simulink model "main_controller_sim"  (R2015a)
settings: Solver=ode45  StartTime=0.0  StopTime=10  FixedStep=1e-3  MaxStep=1e-3  RelTol=1e-3
values from neighbouring files (symbols this model uses):
  A = sys_rand.A    [main_Observer_states.m]
  B = B(:,1:end-1)    [main_Observer_states.m]
  beta = [5657.83678507 -1913.14902282 -932.285352789 348.153105943 2507.13858904 -2140.9545479]    [beta.mat]    (also in main_disturbance_observer.m = inv(delta2)*beta_hat)
  C = [0.617255113405149,0,0,-0.448535555941661,0.134230346538703,1.41932930409004;0.283640603624291,0,2.22808153625508,-1.86462753317668,-1.99763494036701,-0.0116516666362024;0.350975702033898,-0.174162030842294,1.44167650824058,-0.392420914284623,1.30288133017051,-0.392171726620127]    [finding_Y.m]    (also in main_Observer_states.m = sys_rand.C)
  Delta = (eye(n,n)+(-H*CHp+Y*(eye(p,p)-(C*H)*CHp))*C)*B    [main_Observer_states.m]    (also in observer.mat = [-0.0673817558455 0.158220969334 -1.63112233705 -0.121104966)
  Gama = eta*A-X*C    [main_Observer_states.m]    (also in observer.mat = [-0.665415381788 -1.71297839543 -11.0757301234 9.21615917151)
  H = B(:,end)    [main_Observer_states.m]
  Phi = dec2mat(LMISYS,xopt,2)    [main_Observer_states.m]    (also in observer.mat = [2.03974430811 -0.144807404976 -3.64797116197 7.53997403465 )
  theta = theta1+Y*theta2    [main_Observer_states.m]    (also in observer.mat = [-0.848682280391 0.936204937086 2.9983152382 2.21151006385 4)
  Tw = [0.110610315069 0.237446821355 -1.7873542646]    [Tw.mat]
  Tx = [0.778503771805 -0.0510386379765 1.1345792671 0.660349965935 0.317918162843 -0.19578141191 0.0703383785316 -0.0293855404701 0.00570882754881 0.572739299383 0.143983654558 -0.291796802072 ... (18 elements, 3x6)]    [Tx.mat]
libraries: simulink x1
settings Model: Creator=p4wp4w  LastModifiedBy=p4wp4w

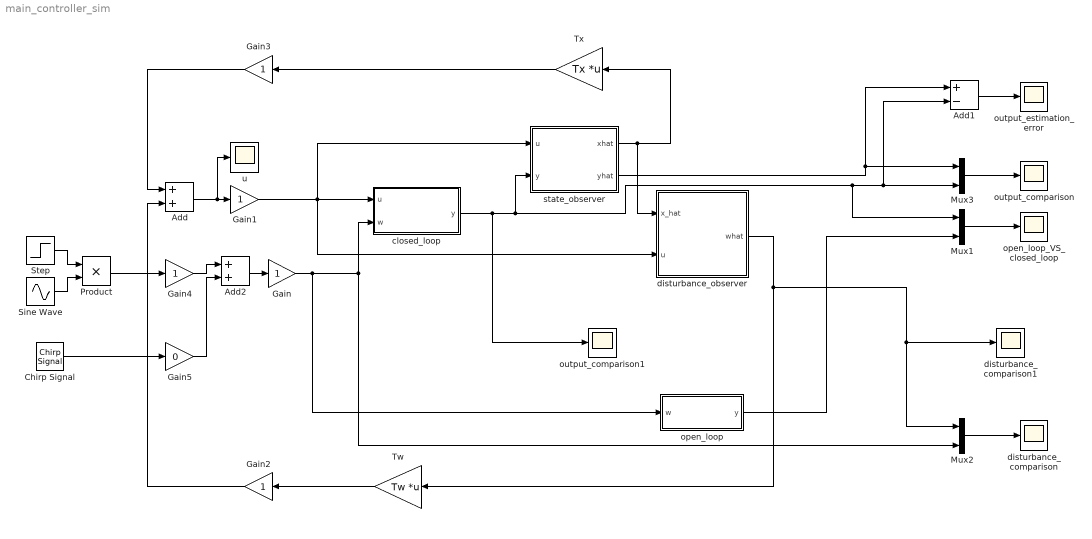
== system main_controller_sim ==
  Add : Sum
  Add1 : Sum  Inputs=+-
  Add2 : Sum
  Chirp Signal : simulink/Sources/Chirp Signal  f1=0.1/2/pi  T=100  f2=1.5/2/pi
  Gain{,1..4} (5 alike) : Gain
  Gain5 : Gain  Gain=0
  Mux1 : Mux  Inputs=2
  Mux2 : Mux  Inputs=2
  Mux3 : Mux  Inputs=2
  Product : Product
  Sine Wave : Sin  Frequency=10  SampleTime=0
  Step : Step  Before=8  After=0  SampleTime=0
  Tw : Gain  Gain=Tw  Multiplication=Matrix(K*u)
  Tx : Gain  Gain=Tx  Multiplication=Matrix(K*u)
  closed_loop : Subsystem
  disturbance_comparison : Scope
      settings: YMin=-15  YMax=15
  disturbance_comparison1 : Scope
      settings: YMin=-15  YMax=15  SaveName=ScopeData6
  disturbance_observer : Subsystem
  open_loop : Subsystem
  open_loop_VS_closed_loop : Scope
      settings: ShowLegends=on  YMin=-5e+22  YMax=3.5e+23  SaveName=ScopeData4
  output_comparison : Scope
      settings: YMin=-0.0024  YMax=-2.1684e-19
  output_comparison1 : Scope
      settings: YMin=-0.0024  YMax=-2.1684e-19  SaveName=ScopeData5
  output_estimation_error : Scope
      settings: YMin=-0.0024  YMax=-2.1684e-19  SaveName=ScopeData3
  state_observer : Subsystem
  u : Scope
      settings: SaveName=ScopeData2
  wires:
  Gain1/1 -> disturbance_observer/2(u), state_observer/1(u), closed_loop/1(u)
  closed_loop/1(y) -> output_comparison1/1, Mux1/1, Add1/2, Mux3/2, state_observer/2(y)
  Mux2/1 -> disturbance_comparison/1
  Mux3/1 -> output_comparison/1
  state_observer/2(yhat) -> Add1/1, Mux3/1
  disturbance_observer/1(what) -> Tw/1, disturbance_comparison1/1, Mux2/1
  Gain/1 -> open_loop/1(w), Mux2/2, closed_loop/2(w)
  state_observer/1(xhat) -> disturbance_observer/1(x_hat), Tx/1
  Add/1 -> u/1, Gain1/1
  Tx/1 -> Gain3/1
  Tw/1 -> Gain2/1
  Gain2/1 -> Add/2
  Gain3/1 -> Add/1
  Add1/1 -> output_estimation_error/1
  open_loop/1(y) -> Mux1/2
  Mux1/1 -> open_loop_VS_closed_loop/1
  Step/1 -> Product/1
  Sine Wave/1 -> Product/2
  Chirp Signal/1 -> Gain5/1
  Product/1 -> Gain4/1
  Add2/1 -> Gain/1
  Gain4/1 -> Add2/1
  Gain5/1 -> Add2/2

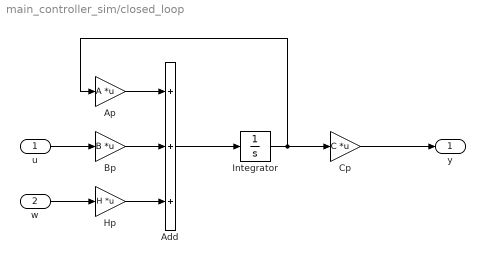
== system main_controller_sim/closed_loop ==
  u : Inport
  w : Inport  Port=2
  Add : Sum  Inputs=+++
  Ap : Gain  Gain=A  Multiplication=Matrix(K*u)
  Bp : Gain  Gain=B  Multiplication=Matrix(K*u)
  Cp : Gain  Gain=C  Multiplication=Matrix(K*u)
  Hp : Gain  Gain=H  Multiplication=Matrix(K*u)
  Integrator : Integrator
  y : Outport
  wires:
  w/1 -> Hp/1
  u/1 -> Bp/1
  Add/1 -> Integrator/1
  Bp/1 -> Add/2
  Integrator/1 -> Cp/1, Ap/1
  Ap/1 -> Add/1
  Hp/1 -> Add/3
  Cp/1 -> y/1

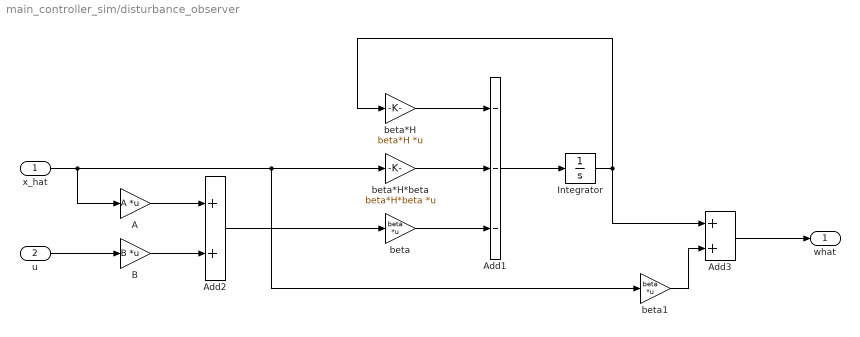
== system main_controller_sim/disturbance_observer ==
  x_hat : Inport
  u : Inport  Port=2
  A : Gain  Gain=A  Multiplication=Matrix(K*u)
  Add1 : Sum  Inputs=---
  Add2 : Sum
  Add3 : Sum
  B : Gain  Gain=B  Multiplication=Matrix(K*u)
  Integrator : Integrator
  beta : Gain  Gain=beta  Multiplication=Matrix(K*u)
  beta*H : Gain  Gain=beta*H  Multiplication=Matrix(K*u)
  beta*H*beta : Gain  Gain=beta*H*beta  Multiplication=Matrix(K*u)
  beta1 : Gain  Gain=beta  Multiplication=Matrix(K*u)
  what : Outport
  wires:
  Add1/1 -> Integrator/1
  beta*H/1 -> Add1/1
  Integrator/1 -> Add3/1, beta*H/1
  beta*H*beta/1 -> Add1/2
  x_hat/1 -> A/1, beta1/1, beta*H*beta/1
  beta/1 -> Add1/3
  A/1 -> Add2/1
  B/1 -> Add2/2
  u/1 -> B/1
  Add2/1 -> beta/1
  beta1/1 -> Add3/2
  Add3/1 -> what/1

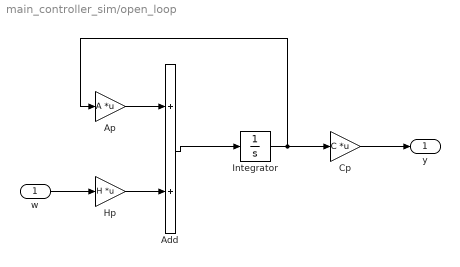
== system main_controller_sim/open_loop ==
  w : Inport
  Add : Sum
  Ap : Gain  Gain=A  Multiplication=Matrix(K*u)
  Cp : Gain  Gain=C  Multiplication=Matrix(K*u)
  Hp : Gain  Gain=H  Multiplication=Matrix(K*u)
  Integrator : Integrator
  y : Outport
  wires:
  Cp/1 -> y/1
  Hp/1 -> Add/2
  Ap/1 -> Add/1
  Integrator/1 -> Ap/1, Cp/1
  Add/1 -> Integrator/1
  w/1 -> Hp/1

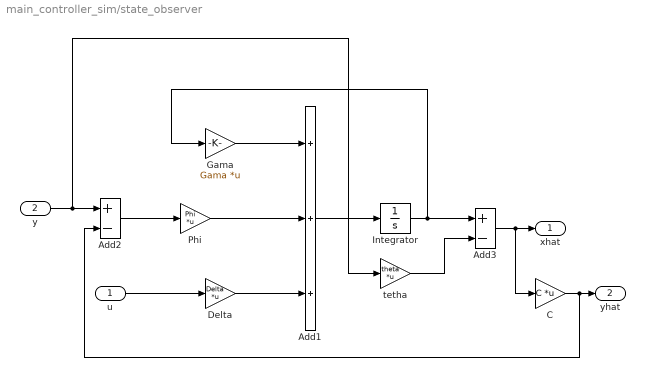
== system main_controller_sim/state_observer ==
  u : Inport
  y : Inport  Port=2
  Add1 : Sum  Inputs=+++
  Add2 : Sum  Inputs=+-
  Add3 : Sum  Inputs=+-
  C : Gain  Gain=C  Multiplication=Matrix(K*u)
  Delta : Gain  Gain=Delta  Multiplication=Matrix(K*u)
  Gama : Gain  Gain=Gama  Multiplication=Matrix(K*u)
  Integrator : Integrator
  Phi : Gain  Gain=Phi  Multiplication=Matrix(K*u)
  tetha : Gain  Gain=theta  Multiplication=Matrix(K*u)
  xhat : Outport
  yhat : Outport  Port=2
  wires:
  y/1 -> tetha/1, Add2/1
  C/1 -> Add2/2, yhat/1
  Add1/1 -> Integrator/1
  Gama/1 -> Add1/1
  Integrator/1 -> Gama/1, Add3/1
  Phi/1 -> Add1/2
  Add2/1 -> Phi/1
  u/1 -> Delta/1
  Delta/1 -> Add1/3
  tetha/1 -> Add3/2
  Add3/1 -> C/1, xhat/1
